simulink library "CtrlIOLib"  (R2022b)
settings: Solver=VariableStepAuto  StartTime=0.0  StopTime=10.0  RelTol=1e-3
libraries: RTC x1
settings Model: Creator=mp55777  LastModifiedBy=mp55777

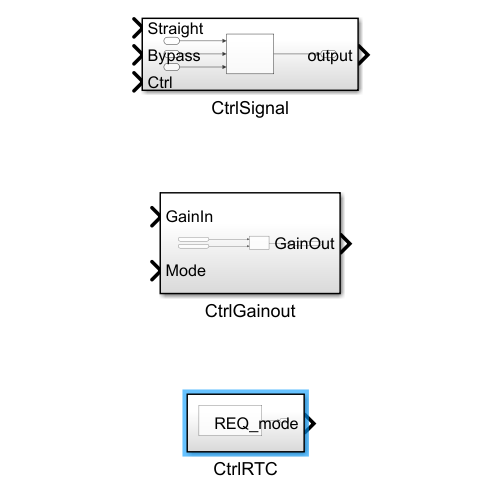
[thumbnail: Simulink's stored preview of the top-level diagram]
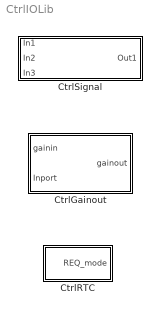
== system CtrlIOLib ==
  CtrlGainout : Subsystem
  CtrlRTC : Subsystem
  CtrlSignal : Subsystem

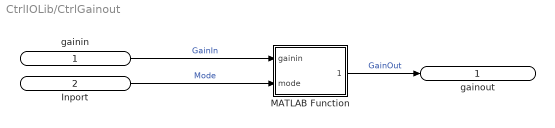
== system CtrlIOLib/CtrlGainout ==
  gainin : Inport
  Inport : Inport  Port=2
  MATLAB Function : MATLAB Function  TreatAsAtomicUnit=on
  gainout : Outport
  wires:
  MATLAB Function/1(gainout) -> gainout/1  "GainOut"
  gainin/1 -> MATLAB Function/1(gainin)  "GainIn"
  Inport/1 -> MATLAB Function/2(mode)  "Mode"

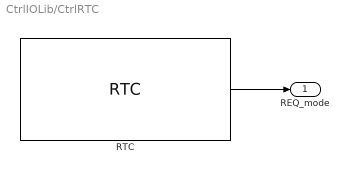
== system CtrlIOLib/CtrlRTC ==
  RTC : RTC/RTC  REQ_Priority=RTC_Mask.NormalPriority  RequestAtInit=off  EnableRequest=off  REQElemName1=mode  REQElemType1=int32  REQElemWidth1=1  REQElemInitial1=[1]  REQElemType2=uint32  REQElemWidth2=1  REQElemInitial2=[]  REQElemType3=uint32  REQElemWidth3=1  REQElemInitial3=[]  REQElemType4=uint32  REQElemWidth4=1  REQElemInitial4=[]  REQElemType5=uint32  REQElemWidth5=1  REQElemInitial5=[]  REQElemType6=uint32  REQElemWidth6=1  REQElemInitial6=[]  REQElemType7=uint32  REQElemWidth7=1  REQElemInitial7=[]  REQElemType8=uint32  REQElemWidth8=1  REQElemInitial8=[]  REQElemType9=uint32  REQElemWidth9=1  REQElemInitial9=[]  REQElemType10=uint32  REQElemWidth10=1  REQElemInitial10=[]  EnableResponse=off  EnableRSP_StatusIn=off  RSPElemType1=uint32  RSPElemWidth1=1  RSPElemType2=uint32  RSPElemWidth2=1  RSPElemType3=uint32  RSPElemWidth3=1  RSPElemType4=uint32  RSPElemWidth4=1  RSPElemType5=uint32  RSPElemWidth5=1  RSPElemType6=uint32  RSPElemWidth6=1  RSPElemType7=uint32  RSPElemWidth7=1  RSPElemType8=uint32  RSPElemWidth8=1  RSPElemType9=uint32  RSPElemWidth9=1  RSPElemType10=uint32  RSPElemWidth10=1  EnableNotification=off  EnableNTF_PrepTrig=off  NTFElemType1=uint32  NTFElemWidth1=1  NTFElemType2=uint32  NTFElemWidth2=1  NTFElemType3=uint32  NTFElemWidth3=1  NTFElemType4=uint32  NTFElemWidth4=1  NTFElemType5=uint32  NTFElemWidth5=1  NTFElemType6=uint32  NTFElemWidth6=1  NTFElemType7=uint32  NTFElemWidth7=1  NTFElemType8=uint32  NTFElemWidth8=1  NTFElemType9=uint32  NTFElemWidth9=1  NTFElemType10=uint32  NTFElemWidth10=1  MaskMessageName=Ctrl
      settings: SourceProductName=Bose Talaria
  REQ_mode : Outport
  wires:
  RTC/1 -> REQ_mode/1

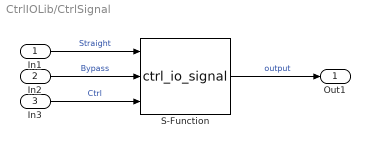
== system CtrlIOLib/CtrlSignal ==
  In1 : Inport  OutDataTypeStr=single
  In2 : Inport  Port=2  OutDataTypeStr=single
  In3 : Inport  Port=3
  S-Function : S-Function  FunctionName=ctrl_io_signal  SFunctionDeploymentMode=off  EnableBusSupport=off
  Out1 : Outport  OutDataTypeStr=single
  wires:
  In1/1 -> S-Function/1  "Straight"
  S-Function/1 -> Out1/1  "output"
  In2/1 -> S-Function/2  "Bypass"
  In3/1 -> S-Function/3  "Ctrl"

== matlab function CtrlIOLib/CtrlGainout/MATLAB Function ==
  data: gainin input; gainout output; mode input
function gainout = fcn(gainin,mode)
    gainout = gainin;
    if (mode == 0)
        gainout(1:end) = 0;
    elseif (mode < 0)
        gainout(1:end) = 1;
    end
